simulink model "vertical_dynamics_vehicle"  (R2025a)
settings: Solver=FixedStepAuto  StartTime=0.0  StopTime=T_sim  FixedStep=T_abt  RelTol=1e-3
values from neighbouring files (symbols this model uses):
  b = 1.4    [vertical_dynamics_kf.m]
  dFh = 2000    [vertical_dynamics_kf.m]
  dFv = 1500    [vertical_dynamics_kf.m]
  dPhi_0 = 0    [vertical_dynamics_kf.m]
  dR = 250    [vertical_dynamics_kf.m]
  dTheta_0 = 0    [vertical_dynamics_kf.m]
  dz1_0 = 0    [vertical_dynamics_kf.m]
  dz2_0 = 0    [vertical_dynamics_kf.m]
  dz3_0 = 0    [vertical_dynamics_kf.m]
  dz4_0 = 0    [vertical_dynamics_kf.m]
  dz5_0 = 0    [vertical_dynamics_kf.m]
  Jphi = 500    [vertical_dynamics_kf.m]
  Jtheta = 2000    [vertical_dynamics_kf.m]
  kFh = 2200    [vertical_dynamics_kf.m]
  kFv = 2500    [vertical_dynamics_kf.m]
  kR = 100000    [vertical_dynamics_kf.m]
  lh = 1.8    [vertical_dynamics_kf.m]
  lv = 1.9    [vertical_dynamics_kf.m]
  m1 = 50    [vertical_dynamics_kf.m]
  m2 = 50    [vertical_dynamics_kf.m]
  m3 = 50    [vertical_dynamics_kf.m]
  m4 = 50    [vertical_dynamics_kf.m]
  m5 = 1200    [vertical_dynamics_kf.m]
  P_0 = Q    [vertical_dynamics_kf.m]
  Phi_0 = 0    [vertical_dynamics_kf.m]
  Q = diag([sigma_z^2,sigma_z^2,sigma_z^2,sigma_z^2,sigma_z^2,sigma_phi^2,sigma_theta^2,    sigma_dz^2,sigma_dz^2,sigma_dz^2,sigma_dz^2,sigma_dz^2,sigma_dphi^2,sigma_dtheta^2 ])*T_abt^2    [vertical_dynamics_kf.m]
  R = diag([sigma_mz^2,sigma_mz^2,sigma_mz^2,sigma_mz^2,sigma_mz^2,sigma_mphi^2,sigma_mtheta^2])    [vertical_dynamics_kf.m]
  seed = randi(1000,3,1)    [vertical_dynamics_kf.m]
  sigma_dphi = 1.6    [vertical_dynamics_kf.m]
  sigma_dtheta = 1.3    [vertical_dynamics_kf.m]
  sigma_dz = 1.1    [vertical_dynamics_kf.m]
  sigma_mphi = 0.2    [vertical_dynamics_kf.m]
  sigma_mtheta = 0.1    [vertical_dynamics_kf.m]
  sigma_mz = 0.1    [vertical_dynamics_kf.m]
  sigma_phi = 1.2    [vertical_dynamics_kf.m]
  sigma_theta = 1.7    [vertical_dynamics_kf.m]
  sigma_z = 1.5    [vertical_dynamics_kf.m]
  T_abt = 0.01    [vertical_dynamics_kf.m]
  Theta_0 = 0    [vertical_dynamics_kf.m]
  x_0 = [z1_0;z2_0;z3_0;z4_0;z5_0;Phi_0;Theta_0;dz1_0;dz2_0;dz3_0;dz4_0;dz5_0;dPhi_0;dTheta_0]    [vertical_dynamics_kf.m]
  z1_0 = 0    [vertical_dynamics_kf.m]
  z2_0 = 0    [vertical_dynamics_kf.m]
  z3_0 = 0    [vertical_dynamics_kf.m]
  z4_0 = 0    [vertical_dynamics_kf.m]
  z5_0 = 0    [vertical_dynamics_kf.m]
(part 2 of 2)

== matlab function vertical_dynamics_vehicle/Kalman_Filter ==
  settings: updateMethod=DISCRETE
  data: u input; x output; y input; kFv parameter; kR parameter; kFh parameter; dR parameter; dFv parameter; dFh parameter; m1 parameter; m2 parameter; m3 parameter; m4 parameter; m5 parameter; Jphi parameter; Jtheta parameter; b parameter; lv parameter; lh parameter; R parameter; Q parameter; P_0 parameter; x_0 parameter; T_abt parameter
function x = kalman_filter(u, y, kFv, kR, kFh, dR, dFv, dFh, m1, m2, m3, m4, m5, Jphi, Jtheta, b, lv, lh, R, Q, P_0, x_0, T_abt)
% R ist die Kovarianzmatrix für das Messrauschen.
% Q ist die Kovarianzmatrix für das Prozessrauschen.k

persistent x_est P_est K
if isempty(x_est)
   x_est = x_0;
   P_est = P_0;
end

%% Discrete Kalman filter time update equations

x = x_est;

% Modellgleichungen in Matrizenform  
A_c = [0                0               0                0               0                         0                        0                              1                0               0                0               0                         0                        0;
       0                0               0                0               0                         0                        0                              0                1               0                0               0                         0                        0;
       0                0               0                0               0                         0                        0                              0                0               1                0               0                         0                        0;
       0                0               0                0               0                         0                        0                              0                0               0                1               0                         0                        0;
       0                0               0                0               0                         0                        0                              0                0               0                0               1                         0                        0;  
       0                0               0                0               0                         0                        0                              0                0               0                0               0                         1                        0;
       0                0               0                0               0                         0                        0                              0                0               0                0               0                         0                        1;
       -(kR+kFv)/m1     0               0                0               kFv/m1                    -b*kFv/(2*m1)            lv*kFv/m1                      -(dR+dFv)/m1     0               0                0               dFv/m1                    -b*dFv/(2*m1)            lv*dFv/m1;
       0                -(kR+kFv)/m2    0                0               kFv/m2                    b*kFv/(2*m2)             lv*kFv/m2                      0                -(dR+dFv)/m2    0                0               dFv/m2                    b*dFv/(2*m2)             lv*dFv/m2;
       0                0               -(kR+kFh)/m3     0               kFh/m3                    -b*kFh/(2*m3)            -lh*kFh/m3                     0                0               -(dR+dFh)/m3     0               dFh/m3                    -b*dFh/(2*m3)            -lh*dFh/m3;
       0                0               0                -(kR+kFh)/m4    kFh/m4                    b*kFh/(2*m4)             -lh*kFh/m4                     0                0               0                -(dR+dFh)/m4    dFh/m4                    b*dFh/(2*m4)             -lh*dFh/m4;
       kFv/m5           kFv/m5          kFh/m5           kFh/m5          -2*(kFv+kFh)/m5           0                        2*(kFh*lh-kFv*lv)/m5           dFv/m5           dFv/m5          dFh/m5           dFh/m5          -2*(dFv+dFh)/m5           0                        2*(dFh*lh-dFv*lv)/m5;
       -b*kFv/(2*Jphi)  b*kFv/(2*Jphi)  -b*kFh/(2*Jphi)  b*kFh/(2*Jphi)  0                         -b^2*(kFh+kFv)/(2*Jphi)  0                              -b*dFv/(2*Jphi)  b*dFv/(2*Jphi)  -b*dFh/(2*Jphi)  b*dFh/(2*Jphi)  0                         -b^2*(dFh+dFv)/(2*Jphi)  0;
       lv*kFv/Jtheta    lv*kFv/Jtheta   -lh*kFh/Jtheta   -lh*kFh/Jtheta  2*(kFh*lh-kFv*lv)/Jtheta  0                        -2*(lv^2*kFv+lh^2*kFh)/Jtheta  lv*dFv/Jtheta    lv*dFv/Jtheta   -lh*dFh/Jtheta   -lh*dFh/Jtheta  2*(kFh*lh-kFv*lv)/Jtheta  0                       -2*(lv^2*dFv+lh^2*dFh)/Jtheta]; 

B_temp = zeros(7,8);
B_c = [B_temp;
       kR/m1  0      0      0      dR/m1  0      0      0;
       0      kR/m2  0      0      0      dR/m2  0      0;
       0      0      kR/m3  0      0      0      dR/m3  0;
       0      0      0      kR/m4  0      0      0      dR/m4;
       0      0      0      0      0      0      0      0;
       0      0      0      0      0      0      0      0;
       0      0      0      0      0      0      0      0]; 
  
% Ad   = diag([ones(1,14)]) + T_abt * A_c;      % Umrechnung in zeitdiskrete Form
Ad = expm(A_c * T_abt);
Bd   = T_abt * B_c;                              % Umrechnung in zeitdiskrete Form


x_ = Ad * x + Bd * u;

C = [1  0  0  0  0  0  0  0  0  0  0  0  0  0;
     0  1  0  0  0  0  0  0  0  0  0  0  0  0;
     0  0  1  0  0  0  0  0  0  0  0  0  0  0;
     0  0  0  1  0  0  0  0  0  0  0  0  0  0;
     0  0  0  0  1  0  0  0  0  0  0  0  0  0;
     0  0  0  0  0  1  0  0  0  0  0  0  0  0;
     0  0  0  0  0  0  1  0  0  0  0  0  0  0];
 

%% Discrete Kalman filter measurement update equations
P_  = Ad * P_est * Ad' + Q;
K   = P_ * C'/( C * P_ * C' + R);
x   = x_ +  K * ( y - C * x_);
% P_est  = P_ - K *( C * P_ * C' + R)* K';
P_est = (eye(14) - K*C) * P_ * (eye(14) - K*C)' + K*R*K'; % Joseph stabilized form
x_est  = x;
y_err = y - C * x_;
